simulink model "lfc2"  (R2024a)
settings: Solver=VariableStepAuto  StartTime=0.0  StopTime=20  FixedStep=1e-6  RelTol=1e-3
settings Model: Creator=farza  LastModifiedBy=farza

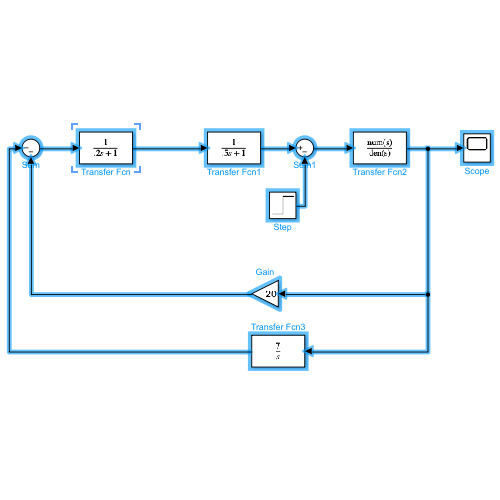
[thumbnail: Simulink's stored preview of the top-level diagram]
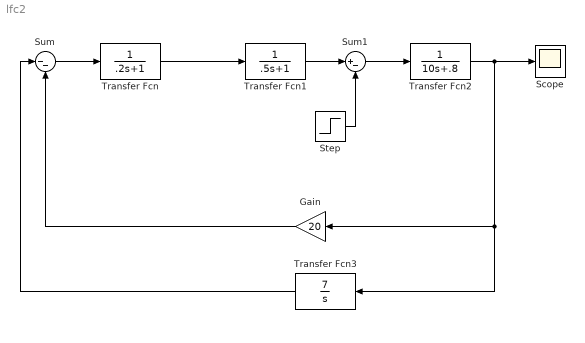
== system lfc2 ==
  Gain : Gain  Gain=20
  Scope : Scope
  Step : Step  After=.2  SampleTime=0
  Sum : Sum  Inputs=|--
  Sum1 : Sum  Inputs=|+-
  Transfer Fcn : TransferFcn  Denominator=[.2 1]
  Transfer Fcn1 : TransferFcn  Denominator=[.5 1]
  Transfer Fcn2 : TransferFcn  Denominator=[10 .8]
  Transfer Fcn3 : TransferFcn  Numerator=[7]  Denominator=[1 0]
  wires:
  Sum/1 -> Transfer Fcn/1
  Gain/1 -> Sum/2
  Transfer Fcn/1 -> Transfer Fcn1/1
  Transfer Fcn1/1 -> Sum1/1
  Sum1/1 -> Transfer Fcn2/1
  Step/1 -> Sum1/2
  Transfer Fcn2/1 -> Transfer Fcn3/1, Gain/1, Scope/1
  Transfer Fcn3/1 -> Sum/1
